simulink model "SecondCOMController"  (Simulink 7.9)
settings: Solver=ode45  StartTime=0.0  StopTime=inf  RelTol=1e-3
libraries: simulink_extras x1, utility x1, dspmtrx3 x1, simulink x1
settings Model: Creator=jorhabib  LastModifiedBy=jorhabib

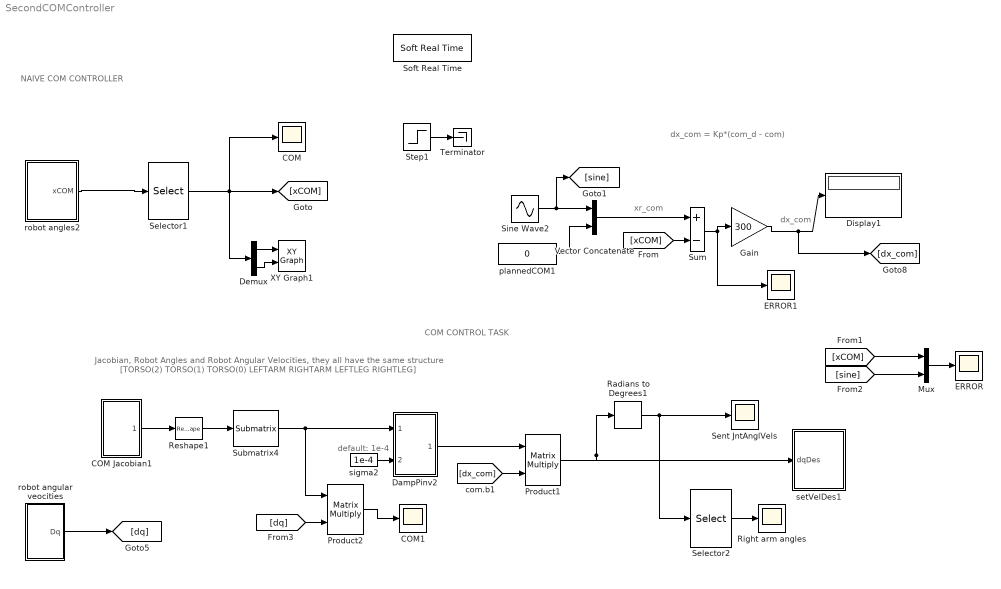
== system SecondCOMController ==
  note: xr_com
  note: dx_com
  note: COM CONTROL TASK
  note: NAIVE COM CONTROLLER
  note: dx_com = Kp*(com_d - com)
  note: default: 1e-4
  note: Jacobian, Robot Angles and Robot Angular Velocities, they all have the same structure
      | [TORSO(2)  TORSO(1)  TORSO(0)    LEFTARM    RIGHTARM    LEFTLEG    RIGHTLEG]
  COM : Scope
      settings: TimeRange=50  YMin=-0.1  YMax=0.175  SaveName=ScopeData4
  COM Jacobian1 : Subsystem
  COM1 : Scope
      settings: TimeRange=50  YMin=-0.00015  YMax=0.0001  SaveName=ScopeData3
  DampPinv2 : Subsystem  mask{tol=1e-4}
      mask prompts: tol "Tolerance"
  Demux : Demux  Outputs=2
  Display1 : Display
  ERROR : Scope
      settings: TimeRange=40  YMin=-0.15  YMax=0.275  SaveName=ScopeData2
  ERROR1 : Scope
      settings: TimeRange=200  YMin=-0.125  YMax=0.175  SaveName=ScopeData5
  Gain : Gain  Gain=300
  Mux : Mux  Inputs=2
  Product1 : Product  Multiplication=Matrix(*)  RndMeth=Zero
  Product2 : Product  Multiplication=Matrix(*)  RndMeth=Zero
  Radians to Degrees1 : simulink_extras/Transformations/Radians to Degrees
  Reshape1 : Reshape  OutputDimensionality=Customize  OutputDimensions=[6,31]
  Right arm angles : Scope
      settings: YMin=-35  YMax=30
  Selector1 : Selector  IndexMode=Zero-based  InputPortWidth=7  IndexOptions=Index vector (dialog)  Indices=[0:1]  OutputSizes=1
  Selector2 : Selector  IndexMode=Zero-based  InputPortWidth=25  IndexOptions=Index vector (dialog)  Indices=[7:11]  OutputSizes=1
  Sent JntAnglVels : Scope
      settings: YMin=-35  YMax=30
  Sine Wave2 : Sin  Amplitude=0.05  Bias=0.0244  Frequency=0.1
  Soft Real Time : utility/Soft Real Time  x=0.02
  Step1 : Step  Time=3  Before=0.024  After=0.05  SampleTime=0
  Submatrix4 : dspmtrx3/Submatrix  RowSpan=Range of rows  RowStartMode=First  RowStartIndex=1  RowEndMode=Index  RowEndIndex=2  ColSpan=Range of columns  ColStartMode=Index  ColStartIndex=7  ColEndMode=Last  ColEndIndex=6
  Sum : Sum  Inputs=+-
  Terminator : Terminator
  Vector Concatenate : Concatenate
  XY Graph1 : simulink/Sinks/XY Graph  xmin=-0.05  xmax=0.05  ymin=-0.05  ymax=0.05  st=-1
  plannedCOM1 : Constant  Value=0  SampleTime=0.05
  robot angles2 : Subsystem
  robot angular veocities : Subsystem
  setVelDes1 : Subsystem
  sigma2 : Constant  Value=1e-4
  wires:
  Vector Concatenate/1 -> Sum/1
  [xCOM] -> Sum/2
  Sum/1 -> Gain/1, ERROR1/1
  Selector1/1 -> [xCOM], Demux/1, COM/1
  robot angles2/1(xCOM) -> Selector1/1
  Sine Wave2/1 -> Vector Concatenate/1, [sine]
  plannedCOM1/1 -> Vector Concatenate/2
  COM Jacobian1/1(Jacobian) -> Reshape1/1
  Reshape1/1 -> Submatrix4/1
  sigma2/1 -> DampPinv2/2(sigma)
  Submatrix4/1 -> DampPinv2/1(mat), Product2/1
  DampPinv2/1(DPinv) -> Product1/1
  [dx_com] -> Product1/2
  Product1/1 -> Radians to Degrees1/1, setVelDes1/1(dqDes)
  Radians to Degrees1/1 -> Sent JntAnglVels/1, Selector2/1
  Gain/1 -> Display1/1, [dx_com]
  Selector2/1 -> Right arm angles/1
  Demux/1 -> XY Graph1/1
  Demux/2 -> XY Graph1/2
  Mux/1 -> ERROR/1
  [xCOM] -> Mux/1
  [sine] -> Mux/2
  Step1/1 -> Terminator/1
  [dq] -> Product2/2
  Product2/1 -> COM1/1
  robot angular veocities/1(Dq) -> [dq]

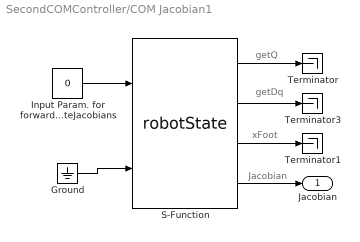
== system SecondCOMController/COM Jacobian1 ==
  note: getDq
  note: xFoot
  note: getQ
  note: Jacobian
  Ground : Ground
  "Input Param. for forwardKinematics and  computeJacobians " : Constant  Value=0  OutDataTypeStr=int8
  S-Function : S-Function  FunctionName=robotState  Parameters=val,robotname,localname  EnableBusSupport=off  mask{val=3, robotname='icubSim', localname='robotState'}
      mask prompts: val "Value"; robotname "Robot Name (icub - icubSim)"; localname "Module Name"
  Terminator : Terminator
  Terminator1 : Terminator
  Terminator3 : Terminator
  Jacobian : Outport
  wires:
  Ground/1 -> S-Function/2
  S-Function/2 -> Terminator3/1
  S-Function/1 -> Terminator/1
  S-Function/3 -> Terminator1/1
  "Input Param. for forwardKinematics and  computeJacobians "/1 -> S-Function/1
  S-Function/4 -> Jacobian/1

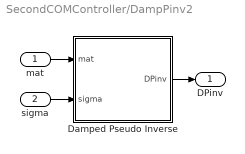
== system SecondCOMController/DampPinv2 ==
  mat : Inport
  sigma : Inport  Port=2
  Damped Pseudo Inverse : MATLAB Function  TreatAsAtomicUnit=on
  DPinv : Outport
  wires:
  sigma/1 -> Damped Pseudo Inverse/2(sigma)
  Damped Pseudo Inverse/1(DPinv) -> DPinv/1
  mat/1 -> Damped Pseudo Inverse/1(mat)

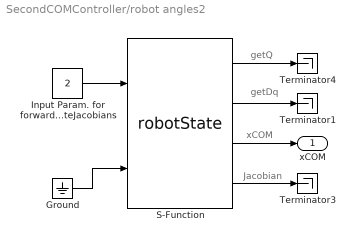
== system SecondCOMController/robot angles2 ==
  note: getDq
  note: xCOM
  note: getQ
  note: Jacobian
  Ground : Ground
  "Input Param. for forwardKinematics and  computeJacobians " : Constant  Value=2  OutDataTypeStr=int8
  S-Function : S-Function  FunctionName=robotState  Parameters=val,robotname,localname  EnableBusSupport=off  mask{val=2, robotname='icubSim', localname='robotState'}
      mask prompts: val "Value"; robotname "Robot Name (icub - icubSim)"; localname "Module Name"
  Terminator1 : Terminator
  Terminator3 : Terminator
  Terminator4 : Terminator
  xCOM : Outport
  wires:
  Ground/1 -> S-Function/2
  S-Function/2 -> Terminator1/1
  S-Function/1 -> Terminator4/1
  S-Function/3 -> xCOM/1
  "Input Param. for forwardKinematics and  computeJacobians "/1 -> S-Function/1
  S-Function/4 -> Terminator3/1

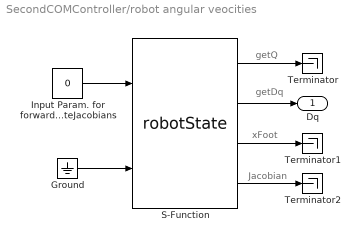
== system SecondCOMController/robot angular veocities ==
  note: Jacobian
  note: getQ
  note: xFoot
  note: getDq
  Ground : Ground
  "Input Param. for forwardKinematics and  computeJacobians " : Constant  Value=0  OutDataTypeStr=int8
  S-Function : S-Function  FunctionName=robotState  Parameters=val,robotname,localname  EnableBusSupport=off  mask{val=1, robotname='icubSim', localname='robotState'}
      mask prompts: val "Value"; robotname "Robot Name (icub - icubSim)"; localname "Module Name"
  Terminator : Terminator
  Terminator1 : Terminator
  Terminator2 : Terminator
  Dq : Outport
  wires:
  S-Function/4 -> Terminator2/1
  "Input Param. for forwardKinematics and  computeJacobians "/1 -> S-Function/1
  S-Function/3 -> Terminator1/1
  S-Function/1 -> Terminator/1
  S-Function/2 -> Dq/1
  Ground/1 -> S-Function/2

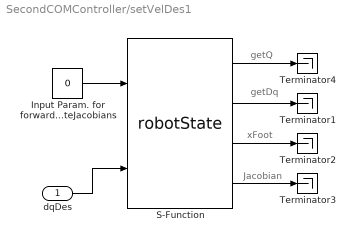
== system SecondCOMController/setVelDes1 ==
  note: getDq
  note: xFoot
  note: getQ
  note: Jacobian
  dqDes : Inport
  "Input Param. for forwardKinematics and  computeJacobians " : Constant  Value=0  OutDataTypeStr=int8
  S-Function : S-Function  FunctionName=robotState  Parameters=val,robotname,localname  EnableBusSupport=off  mask{val=4, robotname='icubSim', localname='robotState'}
      mask prompts: val "Value"; robotname "Robot Name (icub - icubSim)"; localname "Module Name"
  Terminator{1..4} (4 alike) : Terminator
  wires:
  dqDes/1 -> S-Function/2
  S-Function/2 -> Terminator1/1
  S-Function/1 -> Terminator4/1
  S-Function/3 -> Terminator2/1
  "Input Param. for forwardKinematics and  computeJacobians "/1 -> S-Function/1
  S-Function/4 -> Terminator3/1

== matlab function DampPinv2/Damped Pseudo Inverse ==
  data: mat input double; DPinv output double; sigma input double
function DPinv  = fcn(mat,sigma)
% Economy size svd of mat
[U,S,V] = svd(mat,'econ');
% Damped version of S with sigma
S(S>sigma)=S(S>sigma)./((S(S>sigma)).^2+sigma^2);
% Damped pseudoinverse
DPinv = V*pinv(S)*U';
